simulink model "Bioreactor"  (R2014b)
settings: Solver=ode45  StartTime=0.0  StopTime=100  MaxStep=0.5  RelTol=1e-3
libraries: simulink x1
settings Model: Creator=jeff  LastModifiedBy=jeff

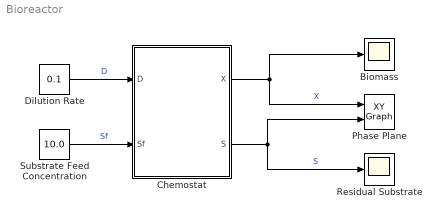
== system Bioreactor ==
  Biomass : Scope
      settings: TimeRange=100  YMin=0
  Chemostat : Subsystem
  Dilution Rate : Constant  Value=0.1
  Phase Plane : simulink/Sinks/XY Graph  xmin=0  xmax=7  ymin=0  ymax=10  st=-1
  Residual Substrate : Scope
      settings: TimeRange=100  YMin=0  YMax=10
  Substrate Feed Concentration : Constant  Value=10.0
  wires:
  Chemostat/1(X) -> Phase Plane/1, Biomass/1  "X"
  Chemostat/2(S) -> Phase Plane/2, Residual Substrate/1  "S"
  Substrate Feed Concentration/1 -> Chemostat/2(Sf)  "Sf"
  Dilution Rate/1 -> Chemostat/1(D)  "D"

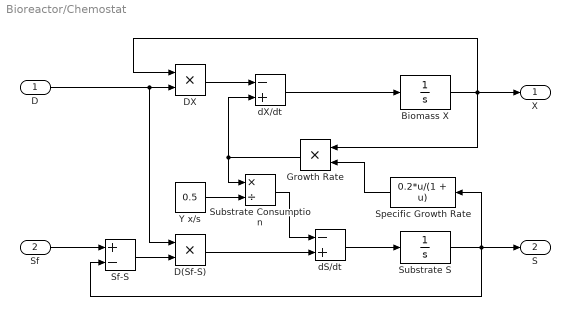
== system Bioreactor/Chemostat ==
  D : Inport
  Sf : Inport  Port=2
  Biomass X : Integrator  InitialCondition=0.5  LimitOutput=on  UpperSaturationLimit=Inf  LowerSaturationLimit=0  ContinuousStateAttributes='biomass'
  D(Sf-S) : Product
  DX : Product
  Growth Rate : Product
  Sf-S : Sum  Inputs=+-
  Specific Growth Rate : Fcn  Expr=0.2*u/(1 + u)
  Substrate Consumption : Product  Inputs=*/
  Substrate S : Integrator  LimitOutput=on  UpperSaturationLimit=Inf  LowerSaturationLimit=0  ContinuousStateAttributes='substrate'
  Y x/s : Constant  Value=0.5
  dS/dt : Sum  Inputs=-+
  dX/dt : Sum  Inputs=-+
  X : Outport
  S : Outport  Port=2
  wires:
  Biomass X/1 -> DX/1, X/1, Growth Rate/1
  DX/1 -> dX/dt/1
  dS/dt/1 -> Substrate S/1
  Substrate Consumption/1 -> dS/dt/1
  Y x/s/1 -> Substrate Consumption/2
  Sf-S/1 -> D(Sf-S)/2
  Specific Growth Rate/1 -> Growth Rate/2
  dX/dt/1 -> Biomass X/1
  D/1 -> D(Sf-S)/1, DX/2
  D(Sf-S)/1 -> dS/dt/2
  Substrate S/1 -> Sf-S/2, S/1, Specific Growth Rate/1
  Growth Rate/1 -> Substrate Consumption/1, dX/dt/2
  Sf/1 -> Sf-S/1
